simulink model "observador_multirate"  (R2012b)
settings: Solver=ode45  StartTime=0.0  StopTime=10  FixedStep=1e-5  MaxStep=1e-4  RelTol=1e-3
values from neighbouring files (symbols this model uses):
  A = [-0.2  0; 1  0]    [enc10_pulsegen0p5.mat]    (also in simulacaoBoaParaDebugar.mat)
  B = [10 0]    [enc10_pulsegen0p5.mat]    (also in simulacaoBoaParaDebugar.mat)
  C = [0 1]    [enc10_pulsegen0p5.mat]    (also in simulacaoBoaParaDebugar.mat)
libraries: simulink x3, Encoder x1
settings Model: Creator=Juliano  LastModifiedBy=Juliano
settings DataIOCC: LimitDataPoints=off

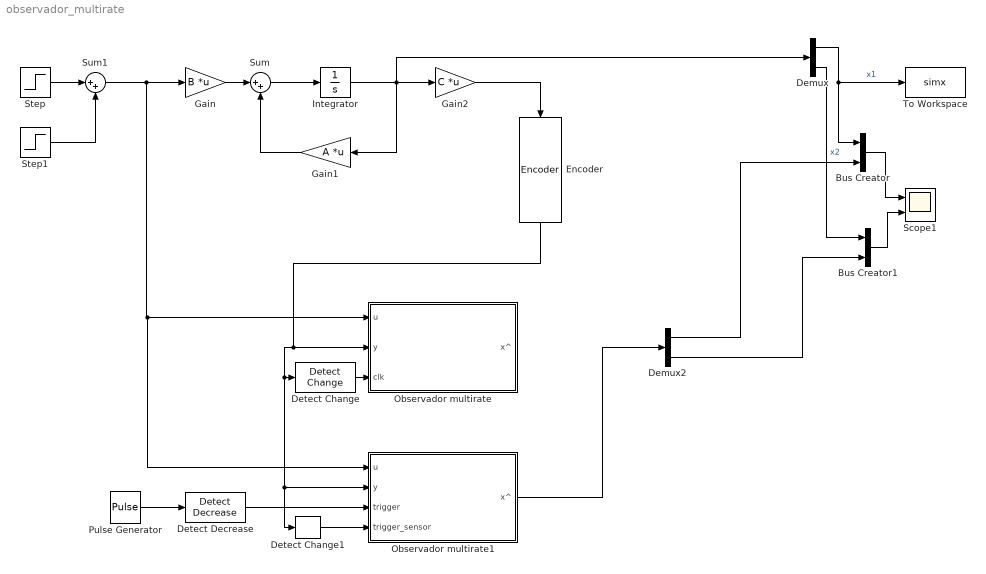
== system observador_multirate ==
  Bus Creator : BusCreator  Inputs=2
  Bus Creator1 : BusCreator  Inputs=2
  Demux : Demux  Outputs=2
  Demux2 : Demux  Outputs=2
  Detect Change : simulink/Logic and Bit Operations/Detect Change  vinit=0  InputProcessing=Inherited  OutDataTypeStr=boolean
  Detect Change1 : simulink/Logic and Bit Operations/Detect Change  vinit=0  InputProcessing=Inherited  OutDataTypeStr=boolean
  Detect Decrease : simulink/Logic and Bit Operations/Detect Decrease  vinit=0.0  InputProcessing=Inherited  OutDataTypeStr=boolean
  Encoder : Encoder/Encoder  Nr=10
  Gain : Gain  Gain=B  Multiplication=Matrix(K*u)
  Gain1 : Gain  Gain=A  Multiplication=Matrix(K*u)
  Gain2 : Gain  Gain=C  Multiplication=Matrix(K*u)
  Integrator : Integrator
  Observador multirate : Subsystem
  Observador multirate1 : Subsystem
  Pulse Generator : DiscretePulseGenerator  PulseType=Time based  Period=0.5  PulseWidth=50
  Scope1 : Scope  NumInputPorts=2
      settings: ShowLegends=on  TimeRange=10  YMin=-750000~-200000  YMax=3.75e+06~1.3e+06
  Step : Step  Time=0  After=20  SampleTime=0
  Step1 : Step  Time=5  After=-40  SampleTime=0
  Sum : Sum  Inputs=|++
  Sum1 : Sum  Inputs=|++
  To Workspace : ToWorkspace  VariableName=simx  SampleTime=-1
  wires:
  Gain/1 -> Sum/1
  Gain1/1 -> Sum/2
  Sum/1 -> Integrator/1
  Integrator/1 -> Demux/1, Gain2/1, Gain1/1
  Step/1 -> Sum1/1
  Step1/1 -> Sum1/2
  Demux/1 -> To Workspace/1, Bus Creator/1  "x1"
  Demux/2 -> Bus Creator1/1  "x2"
  Bus Creator1/1 -> Scope1/2
  Bus Creator/1 -> Scope1/1
  Sum1/1 -> Gain/1, Observador multirate1/1(u), Observador multirate/1(u)
  Encoder/1 -> Observador multirate1/2(y), Detect Change1/1, Detect Change/1, Observador multirate/2(y)
  Demux2/2 -> Bus Creator1/2
  Demux2/1 -> Bus Creator/2
  Detect Change/1 -> Observador multirate/3(clk)
  Gain2/1 -> Encoder/1
  Pulse Generator/1 -> Detect Decrease/1
  Observador multirate1/1(x^) -> Demux2/1
  Detect Change1/1 -> Observador multirate1/4(trigger_sensor)
  Detect Decrease/1 -> Observador multirate1/3(trigger)

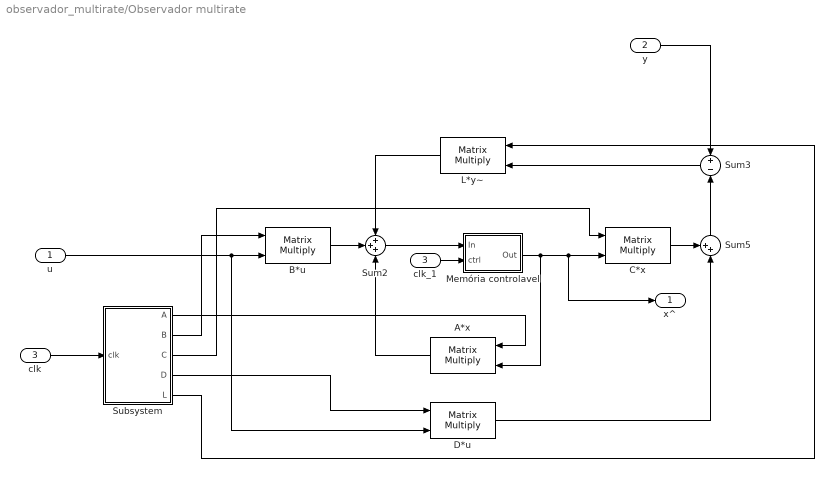
== system observador_multirate/Observador multirate ==
  u : Inport
  y : Inport  Port=2
  clk : Inport  Port=3
  A*x : Product  Multiplication=Matrix(*)  RndMeth=Zero
  B*u : Product  Multiplication=Matrix(*)  RndMeth=Zero
  C*x : Product  Multiplication=Matrix(*)  RndMeth=Zero
  D*u : Product  Multiplication=Matrix(*)  RndMeth=Zero
  L*y~ : Product  Multiplication=Matrix(*)  RndMeth=Zero
  Memória controlavel : Subsystem
  Subsystem : Subsystem
  Sum2 : Sum  Inputs=+++
  Sum3 : Sum  Inputs=+-
  Sum5 : Sum  Inputs=++|
  clk_1 : InportShadow  Port=3
  x^ : Outport
  wires:
  Memória controlavel/1(Out) -> A*x/2, x^/1, C*x/2
  Sum2/1 -> Memória controlavel/1(In)
  B*u/1 -> Sum2/2
  L*y~/1 -> Sum2/1
  C*x/1 -> Sum5/1
  u/1 -> D*u/2, B*u/2
  D*u/1 -> Sum5/2
  y/1 -> Sum3/1
  Sum5/1 -> Sum3/2
  clk/1 -> Subsystem/1(clk)
  A*x/1 -> Sum2/3
  Subsystem/2(B) -> B*u/1
  clk_1/1 -> Memória controlavel/2(ctrl)
  Subsystem/5(L) -> L*y~/1
  Sum3/1 -> L*y~/2
  Subsystem/1(A) -> A*x/1
  Subsystem/4(D) -> D*u/1
  Subsystem/3(C) -> C*x/1

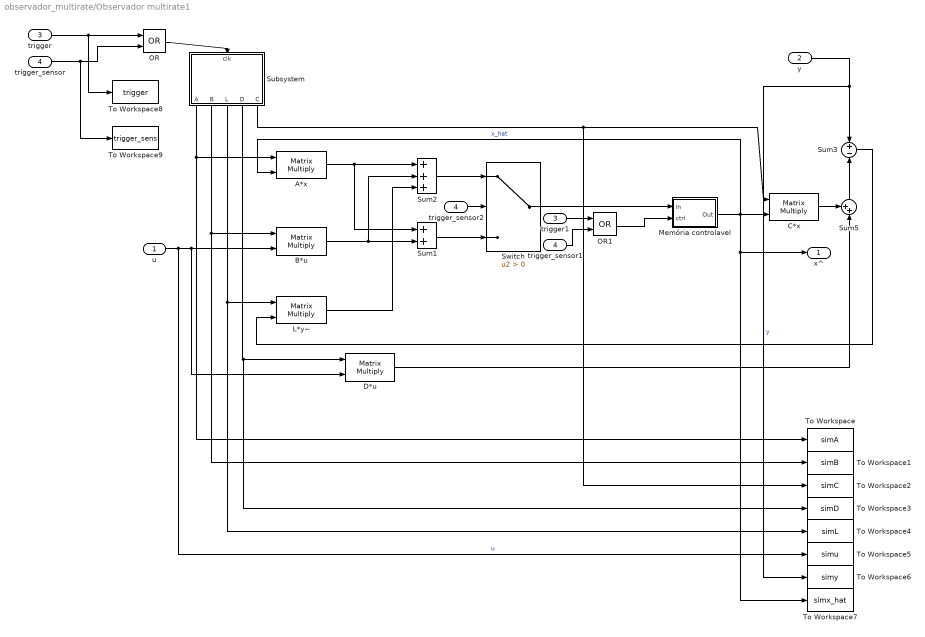
== system observador_multirate/Observador multirate1 ==
  u : Inport
  y : Inport  Port=2
  trigger : Inport  Port=3
  trigger_sensor : Inport  Port=4
  A*x : Product  Multiplication=Matrix(*)  RndMeth=Zero
  B*u : Product  Multiplication=Matrix(*)  RndMeth=Zero
  C*x : Product  Multiplication=Matrix(*)  RndMeth=Zero
  D*u : Product  Multiplication=Matrix(*)  RndMeth=Zero
  L*y~ : Product  Multiplication=Matrix(*)  RndMeth=Zero
  Memória controlavel : Subsystem
  OR : Logic  Operator=OR  AllPortsSameDT=off  OutDataTypeStr=boolean
  OR1 : Logic  Operator=OR  AllPortsSameDT=off  OutDataTypeStr=boolean
  Subsystem : Subsystem
  Sum1 : Sum
  Sum2 : Sum  Inputs=+++
  Sum3 : Sum  Inputs=+-
  Sum5 : Sum  Inputs=++|
  Switch : Switch  Criteria=u2 > Threshold
  To Workspace : ToWorkspace  VariableName=simA  SampleTime=-1
  To Workspace1 : ToWorkspace  VariableName=simB  SampleTime=-1
  To Workspace2 : ToWorkspace  VariableName=simC  SampleTime=-1
  To Workspace3 : ToWorkspace  VariableName=simD  SampleTime=-1
  To Workspace4 : ToWorkspace  VariableName=simL  SampleTime=-1
  To Workspace5 : ToWorkspace  VariableName=simu  SampleTime=-1
  To Workspace6 : ToWorkspace  VariableName=simy  SampleTime=-1
  To Workspace7 : ToWorkspace  VariableName=simx_hat  SampleTime=-1
  To Workspace8 : ToWorkspace  VariableName=trigger  SampleTime=-1
  To Workspace9 : ToWorkspace  VariableName=trigger_sens  SampleTime=-1
  trigger1 : InportShadow  Port=3
  trigger_sensor1 : InportShadow  Port=4
  trigger_sensor2 : InportShadow  Port=4
  x^ : Outport
  wires:
  Memória controlavel/1(Out) -> A*x/2, C*x/2, To Workspace7/1, x^/1  "x_hat"
  C*x/1 -> Sum5/1
  u/1 -> To Workspace5/1, B*u/2, D*u/2  "u"
  D*u/1 -> Sum5/2
  Subsystem/1(A) -> To Workspace/1, A*x/1
  Subsystem/2(B) -> To Workspace1/1, B*u/1
  Subsystem/3(L) -> To Workspace4/1, L*y~/1
  Subsystem/4(D) -> To Workspace3/1, D*u/1
  A*x/1 -> Sum2/1, Sum1/1
  B*u/1 -> Sum2/2, Sum1/2
  Sum2/1 -> Switch/1
  Sum1/1 -> Switch/3
  Switch/1 -> Memória controlavel/1(In)
  Subsystem/5(C) -> To Workspace2/1, C*x/1
  y/1 -> To Workspace6/1, Sum3/1  "y"
  Sum5/1 -> Sum3/2
  Sum3/1 -> L*y~/2
  trigger1/1 -> OR1/1
  trigger_sensor1/1 -> OR1/2
  OR1/1 -> Memória controlavel/2(ctrl)
  trigger/1 -> To Workspace8/1, OR/1
  trigger_sensor/1 -> To Workspace9/1, OR/2
  OR/1 -> Subsystem/1(clk)
  trigger_sensor2/1 -> Switch/2
  L*y~/1 -> Sum2/3

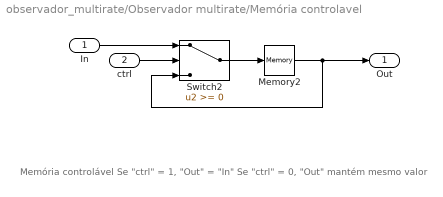
== system observador_multirate/Observador multirate/Memória controlavel ==
  note: Memória controlável
      |
      | Se "ctrl" = 1, "Out" = "In"
      | Se "ctrl" = 0, "Out" mantém mesmo valor
  In : Inport
  ctrl : Inport  Port=2
  Memory2 : Memory
  Switch2 : Switch
  Out : Outport
  wires:
  Switch2/1 -> Memory2/1
  Memory2/1 -> Out/1, Switch2/3
  ctrl/1 -> Switch2/2
  In/1 -> Switch2/1

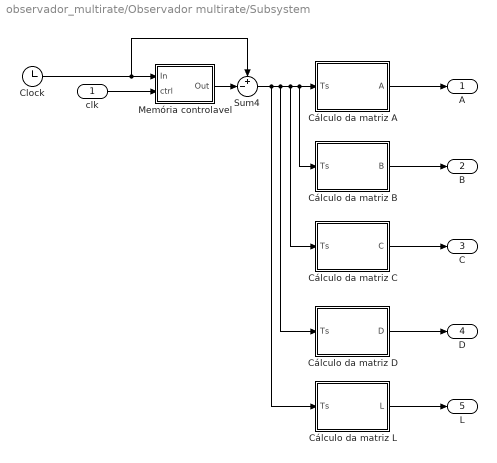
== system observador_multirate/Observador multirate/Subsystem ==
  clk : Inport
  Clock : Clock
  Cálculo da matriz A : MATLAB Function  TreatAsAtomicUnit=on
  Cálculo da matriz B : MATLAB Function  TreatAsAtomicUnit=on
  Cálculo da matriz C : MATLAB Function  TreatAsAtomicUnit=on
  Cálculo da matriz D : MATLAB Function  TreatAsAtomicUnit=on
  Cálculo da matriz L : MATLAB Function  TreatAsAtomicUnit=on
  Memória controlavel : Subsystem
  Sum4 : Sum  Inputs=+-|
  A : Outport
  B : Outport  Port=2
  C : Outport  Port=3
  D : Outport  Port=4
  L : Outport  Port=5
  wires:
  Clock/1 -> Sum4/1, Memória controlavel/1(In)
  Memória controlavel/1(Out) -> Sum4/2
  clk/1 -> Memória controlavel/2(ctrl)
  Sum4/1 -> Cálculo da matriz L/1(Ts), Cálculo da matriz D/1(Ts), Cálculo da matriz C/1(Ts), Cálculo da matriz B/1(Ts), Cálculo da matriz A/1(Ts)
  Cálculo da matriz A/1(A) -> A/1
  Cálculo da matriz B/1(B) -> B/1
  Cálculo da matriz C/1(C) -> C/1
  Cálculo da matriz D/1(D) -> D/1
  Cálculo da matriz L/1(L) -> L/1

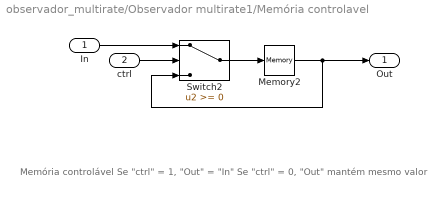
== system observador_multirate/Observador multirate1/Memória controlavel ==
  note: Memória controlável
      |
      | Se "ctrl" = 1, "Out" = "In"
      | Se "ctrl" = 0, "Out" mantém mesmo valor
  In : Inport
  ctrl : Inport  Port=2
  Memory2 : Memory
  Switch2 : Switch
  Out : Outport
  wires:
  Switch2/1 -> Memory2/1
  Memory2/1 -> Out/1, Switch2/3
  ctrl/1 -> Switch2/2
  In/1 -> Switch2/1

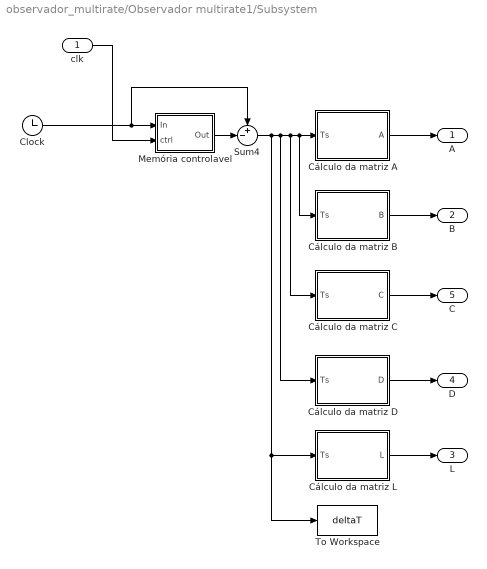
== system observador_multirate/Observador multirate1/Subsystem ==
  clk : Inport
  Clock : Clock
  Cálculo da matriz A : MATLAB Function  TreatAsAtomicUnit=on
  Cálculo da matriz B : MATLAB Function  TreatAsAtomicUnit=on
  Cálculo da matriz C : MATLAB Function  TreatAsAtomicUnit=on
  Cálculo da matriz D : MATLAB Function  TreatAsAtomicUnit=on
  Cálculo da matriz L : MATLAB Function  TreatAsAtomicUnit=on
  Memória controlavel : Subsystem
  Sum4 : Sum  Inputs=+-|
  To Workspace : ToWorkspace  VariableName=deltaT  SampleTime=-1
  A : Outport
  B : Outport  Port=2
  L : Outport  Port=3
  D : Outport  Port=4
  C : Outport  Port=5
  wires:
  Clock/1 -> Sum4/1, Memória controlavel/1(In)
  Memória controlavel/1(Out) -> Sum4/2
  clk/1 -> Memória controlavel/2(ctrl)
  Sum4/1 -> To Workspace/1, Cálculo da matriz L/1(Ts), Cálculo da matriz D/1(Ts), Cálculo da matriz C/1(Ts), Cálculo da matriz B/1(Ts), Cálculo da matriz A/1(Ts)
  Cálculo da matriz A/1(A) -> A/1
  Cálculo da matriz B/1(B) -> B/1
  Cálculo da matriz C/1(C) -> C/1
  Cálculo da matriz D/1(D) -> D/1
  Cálculo da matriz L/1(L) -> L/1

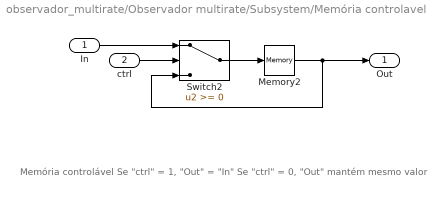
== system observador_multirate/Observador multirate/Subsystem/Memória controlavel ==
  note: Memória controlável
      |
      | Se "ctrl" = 1, "Out" = "In"
      | Se "ctrl" = 0, "Out" mantém mesmo valor
  In : Inport
  ctrl : Inport  Port=2
  Memory2 : Memory
  Switch2 : Switch
  Out : Outport
  wires:
  In/1 -> Switch2/1
  ctrl/1 -> Switch2/2
  Memory2/1 -> Switch2/3, Out/1
  Switch2/1 -> Memory2/1

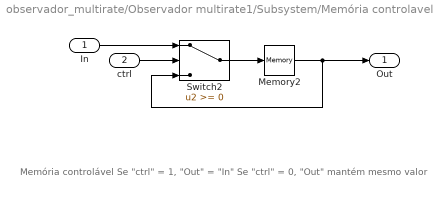
== system observador_multirate/Observador multirate1/Subsystem/Memória controlavel ==
  note: Memória controlável
      |
      | Se "ctrl" = 1, "Out" = "In"
      | Se "ctrl" = 0, "Out" mantém mesmo valor
  In : Inport
  ctrl : Inport  Port=2
  Memory2 : Memory
  Switch2 : Switch
  Out : Outport
  wires:
  In/1 -> Switch2/1
  ctrl/1 -> Switch2/2
  Memory2/1 -> Switch2/3, Out/1
  Switch2/1 -> Memory2/1

== matlab function observador_multirate/Observador multirate/Subsystem/Cálculo da matriz B ==
  data: Ts input; B output
function B = fcn(Ts)
%#codegen

B = [10*Ts ; 0];

== matlab function observador_multirate/Observador multirate/Subsystem/Cálculo da matriz A ==
  data: Ts input; A output
function A = fcn(Ts)
%#codegen

A = [1-0.2*Ts 0 ; Ts 1];

== matlab function observador_multirate/Observador multirate/Subsystem/Cálculo da matriz C ==
  data: Ts input; C output
function C = fcn(Ts)
%#codegen

C = [0 1];

== matlab function observador_multirate/Observador multirate/Subsystem/Cálculo da matriz D ==
  data: Ts input; D output
function D = fcn(Ts)
%#codegen

D = [0];

== matlab function observador_multirate/Observador multirate/Subsystem/Cálculo da matriz L ==
  data: Ts input; L output
function L = fcn(Ts)
%#codegen

L = [-0.18+0.2/Ts+0.04*Ts ; 0.9-0.2*Ts];

== matlab function observador_multirate/Observador multirate1/Subsystem/Cálculo da matriz A ==
  data: Ts input; A output
function A = fcn(Ts)
%#codegen

A = [1-0.2*Ts 0 ; Ts 1];

== matlab function observador_multirate/Observador multirate1/Subsystem/Cálculo da matriz B ==
  data: Ts input; B output
function B = fcn(Ts)
%#codegen

B = [10*Ts ; 0];

== matlab function observador_multirate/Observador multirate1/Subsystem/Cálculo da matriz C ==
  data: Ts input; C output
function C = fcn(Ts)
%#codegen

C = [0 1];

== matlab function observador_multirate/Observador multirate1/Subsystem/Cálculo da matriz D ==
  data: Ts input; D output
function D = fcn(Ts)
%#codegen

D = [0];

== matlab function observador_multirate/Observador multirate1/Subsystem/Cálculo da matriz L ==
  data: Ts input; L output
function L = fcn(Ts)
%#codegen

L = [-0.18+0.2/Ts+0.04*Ts ; 0.9-0.2*Ts];
